simulink model "MSBR_Plant"  (R2021b)
settings: Solver=ode45  StartTime=0.0  StopTime=sim_time  MaxStep=ts_max  RelTol=1e-4
values from neighbouring files (symbols this model uses):
  a_1 = 8.7292e-2/wilson_ratio    (= 0.0087292)    [Whole_Plant_Cool_Pump_Accident_script.m]    (also in Whole_Plant_Fert_Pump_Accident_script.m; Whole_Plant_Fuel_Pump_Accident.m; Whole_Plant_Fuel_Pump_Accident_script.m; Whole_Plant_Reactivity_Accident.m)
  a_2 = 7.3787e-4/wilson_ratio    (= 7.3787e-05)    [Whole_Plant_Cool_Pump_Accident_script.m]    (also in Whole_Plant_Fert_Pump_Accident_script.m; Whole_Plant_Fuel_Pump_Accident.m; Whole_Plant_Fuel_Pump_Accident_script.m; Whole_Plant_Reactivity_Accident.m)
  a_b = 1.656e-5    (= 1.656e-05)    [Whole_Plant_Cool_Pump_Accident_script.m]    (also in Whole_Plant_Fert_Pump_Accident_script.m; Whole_Plant_Fuel_Pump_Accident.m; Whole_Plant_Fuel_Pump_Accident_script.m; Whole_Plant_Reactivity_Accident.m)
  a_f = -8.172e-5    (= -8.172e-05)    [Whole_Plant_Cool_Pump_Accident_script.m]    (also in Whole_Plant_Fert_Pump_Accident_script.m; Whole_Plant_Fuel_Pump_Accident.m; Whole_Plant_Fuel_Pump_Accident_script.m; Whole_Plant_Reactivity_Accident.m)
  a_g = 2.016e-5    (= 2.016e-05)    [Whole_Plant_Cool_Pump_Accident_script.m]    (also in Whole_Plant_Fert_Pump_Accident_script.m; Whole_Plant_Fuel_Pump_Accident.m; Whole_Plant_Fuel_Pump_Accident_script.m; Whole_Plant_Reactivity_Accident.m)
  A_s = pi()*((D_OTSG_i^2)/4) - A_w_OTSG - A_p_OTSG    [Whole_Plant_Cool_Pump_Accident_script.m]    (also in Whole_Plant_Fert_Pump_Accident_script.m; Whole_Plant_Fuel_Pump_Accident.m; Whole_Plant_Fuel_Pump_Accident_script.m; Whole_Plant_Reactivity_Accident.m)
  alpha_co = 316.2    [Whole_Plant_Cool_Pump_Accident_script.m]    (also in Whole_Plant_Fert_Pump_Accident_script.m; Whole_Plant_Fuel_Pump_Accident.m; Whole_Plant_Fuel_Pump_Accident_script.m; Whole_Plant_Reactivity_Accident.m)
  beta = [2.290e-04, 8.320e-04, 7.100e-04, 8.520e-04, 1.710e-04, 1.020e-04]    [Whole_Plant_Cool_Pump_Accident_script.m]    (also in Whole_Plant_Fert_Pump_Accident_script.m; Whole_Plant_Fuel_Pump_Accident.m; Whole_Plant_Fuel_Pump_Accident_script.m; Whole_Plant_Reactivity_Accident.m)
  beta_co = 68.0958    [Whole_Plant_Cool_Pump_Accident_script.m]    (also in Whole_Plant_Fert_Pump_Accident_script.m; Whole_Plant_Fuel_Pump_Accident.m; Whole_Plant_Fuel_Pump_Accident_script.m; Whole_Plant_Reactivity_Accident.m)
  beta_t = sum(beta)    [Whole_Plant_Cool_Pump_Accident_script.m]    (also in Whole_Plant_Fert_Pump_Accident_script.m; Whole_Plant_Fuel_Pump_Accident.m; Whole_Plant_Fuel_Pump_Accident_script.m; Whole_Plant_Reactivity_Accident.m)
  C_nc_X_A_nc = 12.8    [Whole_Plant_Cool_Pump_Accident_script.m]    (also in Whole_Plant_Fert_Pump_Accident_script.m; Whole_Plant_Fuel_Pump_Accident.m; Whole_Plant_Fuel_Pump_Accident_script.m; Whole_Plant_Reactivity_Accident.m)
  C_pcw = 0.0042    [Whole_Plant_Cool_Pump_Accident_script.m]    (also in Whole_Plant_Fert_Pump_Accident_script.m; Whole_Plant_Fuel_Pump_Accident.m; Whole_Plant_Fuel_Pump_Accident_script.m; Whole_Plant_Reactivity_Accident.m)
  C_rh_X_A_rh = 33    [Whole_Plant_Cool_Pump_Accident_script.m]    (also in Whole_Plant_Fert_Pump_Accident_script.m; Whole_Plant_Fuel_Pump_Accident.m; Whole_Plant_Fuel_Pump_Accident_script.m; Whole_Plant_Reactivity_Accident.m)
  C_v = 0.84    [Whole_Plant_Cool_Pump_Accident_script.m]    (also in Whole_Plant_Fert_Pump_Accident_script.m; Whole_Plant_Fuel_Pump_Accident.m; Whole_Plant_Fuel_Pump_Accident_script.m; Whole_Plant_Reactivity_Accident.m)
  ce1 = 1.2471e-07    [Whole_Plant_Cool_Pump_Accident_script.m]    (also in Whole_Plant_Fert_Pump_Accident_script.m; Whole_Plant_Fuel_Pump_Accident.m; Whole_Plant_Fuel_Pump_Accident_script.m; Whole_Plant_Reactivity_Accident.m)
  ce2 = 5.3816e-14    [Whole_Plant_Cool_Pump_Accident_script.m]    (also in Whole_Plant_Fert_Pump_Accident_script.m; Whole_Plant_Fuel_Pump_Accident.m; Whole_Plant_Fuel_Pump_Accident_script.m; Whole_Plant_Reactivity_Accident.m)
  ce3 = 3.3721e-08    [Whole_Plant_Cool_Pump_Accident_script.m]    (also in Whole_Plant_Fert_Pump_Accident_script.m; Whole_Plant_Fuel_Pump_Accident.m; Whole_Plant_Fuel_Pump_Accident_script.m; Whole_Plant_Reactivity_Accident.m)
  Cp_fw = XSteam('Cp_pT',P_set*10,T_fw)/1000    [Whole_Plant_Cool_Pump_Accident_script.m]    (also in Whole_Plant_Fert_Pump_Accident_script.m; Whole_Plant_Fuel_Pump_Accident.m; Whole_Plant_Fuel_Pump_Accident_script.m; Whole_Plant_Reactivity_Accident.m)
  Cp_p = Cp_sec    (= 0.001716588)    [Whole_Plant_Cool_Pump_Accident_script.m]    (also in Whole_Plant_Fert_Pump_Accident_script.m; Whole_Plant_Fuel_Pump_Accident.m; Whole_Plant_Fuel_Pump_Accident_script.m; Whole_Plant_Reactivity_Accident.m)
  Cp_rh = 0.0021520    (= 0.002152)    [Whole_Plant_Cool_Pump_Accident_script.m]    (also in Whole_Plant_Fert_Pump_Accident_script.m; Whole_Plant_Fuel_Pump_Accident.m; Whole_Plant_Fuel_Pump_Accident_script.m; Whole_Plant_Reactivity_Accident.m)
  Cp_s = XSteam('Cp_pT',P_s*10,T_s)/1000    [Whole_Plant_Cool_Pump_Accident_script.m]    (also in Whole_Plant_Fert_Pump_Accident_script.m; Whole_Plant_Fuel_Pump_Accident.m; Whole_Plant_Fuel_Pump_Accident_script.m; Whole_Plant_Reactivity_Accident.m)
  Cp_sc = XSteam('Cp_pT',P_set*10,T_sc2)/1000    [Whole_Plant_Cool_Pump_Accident_script.m]    (also in Whole_Plant_Fert_Pump_Accident_script.m; Whole_Plant_Fuel_Pump_Accident.m; Whole_Plant_Fuel_Pump_Accident_script.m; Whole_Plant_Reactivity_Accident.m)
  Cp_w = 468.992e-6    (= 0.000468992)    [Whole_Plant_Cool_Pump_Accident_script.m]    (also in Whole_Plant_Fert_Pump_Accident_script.m; Whole_Plant_Fuel_Pump_Accident.m; Whole_Plant_Fuel_Pump_Accident_script.m; Whole_Plant_Reactivity_Accident.m)
  D_it = D_ot-2*T_th    (= 0.014147)    [Whole_Plant_Cool_Pump_Accident_script.m]    (also in Whole_Plant_Fert_Pump_Accident_script.m; Whole_Plant_Fuel_Pump_Accident.m; Whole_Plant_Fuel_Pump_Accident_script.m; Whole_Plant_Reactivity_Accident.m)
  D_ot = 0.015875    [Whole_Plant_Cool_Pump_Accident_script.m]    (also in Whole_Plant_Fert_Pump_Accident_script.m; Whole_Plant_Fuel_Pump_Accident.m; Whole_Plant_Fuel_Pump_Accident_script.m; Whole_Plant_Reactivity_Accident.m)
  dHs_dPs = c(1)    [Whole_Plant_Cool_Pump_Accident_script.m]    (also in Whole_Plant_Fert_Pump_Accident_script.m; Whole_Plant_Fuel_Pump_Accident.m; Whole_Plant_Fuel_Pump_Accident_script.m; Whole_Plant_Reactivity_Accident.m)
  eta_hp_isen = 0.861    [Whole_Plant_Cool_Pump_Accident_script.m]    (also in Whole_Plant_Fert_Pump_Accident_script.m; Whole_Plant_Fuel_Pump_Accident.m; Whole_Plant_Fuel_Pump_Accident_script.m; Whole_Plant_Reactivity_Accident.m)
  eta_lp_isen = 0.861    [Whole_Plant_Cool_Pump_Accident_script.m]    (also in Whole_Plant_Fert_Pump_Accident_script.m; Whole_Plant_Fuel_Pump_Accident.m; Whole_Plant_Fuel_Pump_Accident_script.m; Whole_Plant_Reactivity_Accident.m)
  gamma_I = 5.1135e-2    (= 0.051135)    [Whole_Plant_Cool_Pump_Accident_script.m]    (also in Whole_Plant_Fert_Pump_Accident_script.m; Whole_Plant_Fuel_Pump_Accident.m; Whole_Plant_Fuel_Pump_Accident_script.m; Whole_Plant_Reactivity_Accident.m)
  gamma_Xe = 1.1628e-2    (= 0.011628)    [Whole_Plant_Cool_Pump_Accident_script.m]    (also in Whole_Plant_Fert_Pump_Accident_script.m; Whole_Plant_Fuel_Pump_Accident.m; Whole_Plant_Fuel_Pump_Accident_script.m; Whole_Plant_Reactivity_Accident.m)
  H_co0 = 0.149    [Whole_Plant_Cool_Pump_Accident_script.m]    (also in Whole_Plant_Fert_Pump_Accident_script.m; Whole_Plant_Fuel_Pump_Accident.m; Whole_Plant_Fuel_Pump_Accident_script.m; Whole_Plant_Reactivity_Accident.m)
  H_f_co0 = 0.149    [Whole_Plant_Cool_Pump_Accident_script.m]    (also in Whole_Plant_Fert_Pump_Accident_script.m; Whole_Plant_Fuel_Pump_Accident.m; Whole_Plant_Fuel_Pump_Accident_script.m; Whole_Plant_Reactivity_Accident.m)
  H_fg_co0 = 2.35    [Whole_Plant_Cool_Pump_Accident_script.m]    (also in Whole_Plant_Fert_Pump_Accident_script.m; Whole_Plant_Fuel_Pump_Accident.m; Whole_Plant_Fuel_Pump_Accident_script.m; Whole_Plant_Reactivity_Accident.m)
  H_fgrh0 = (XSteam('hV_p', P_s*1e1) - XSteam('hL_p', P_s*1e1))/1e3    [Whole_Plant_Cool_Pump_Accident_script.m]    (also in Whole_Plant_Fert_Pump_Accident_script.m; Whole_Plant_Fuel_Pump_Accident.m; Whole_Plant_Fuel_Pump_Accident_script.m; Whole_Plant_Reactivity_Accident.m)
  H_frh0 = XSteam('hL_p', P_s*1e1)/1e3    [Whole_Plant_Cool_Pump_Accident_script.m]    (also in Whole_Plant_Fert_Pump_Accident_script.m; Whole_Plant_Fuel_Pump_Accident.m; Whole_Plant_Fuel_Pump_Accident_script.m; Whole_Plant_Reactivity_Accident.m)
  h_fwh1 = 0.5927    [Whole_Plant_Cool_Pump_Accident_script.m]    (also in Whole_Plant_Fert_Pump_Accident_script.m; Whole_Plant_Fuel_Pump_Accident.m; Whole_Plant_Fuel_Pump_Accident_script.m; Whole_Plant_Reactivity_Accident.m)
  H_fwh10 = 0.46009    [Whole_Plant_Cool_Pump_Accident_script.m]    (also in Whole_Plant_Fert_Pump_Accident_script.m; Whole_Plant_Fuel_Pump_Accident.m; Whole_Plant_Fuel_Pump_Accident_script.m; Whole_Plant_Reactivity_Accident.m)
  h_fwh2 = 1.230803    [Whole_Plant_Cool_Pump_Accident_script.m]    (also in Whole_Plant_Fert_Pump_Accident_script.m; Whole_Plant_Fuel_Pump_Accident.m; Whole_Plant_Fuel_Pump_Accident_script.m; Whole_Plant_Reactivity_Accident.m)
  H_fwh20 = 0.6784    [Whole_Plant_Cool_Pump_Accident_script.m]    (also in Whole_Plant_Fert_Pump_Accident_script.m; Whole_Plant_Fuel_Pump_Accident.m; Whole_Plant_Fuel_Pump_Accident_script.m; Whole_Plant_Reactivity_Accident.m)
  H_grh0 = 2.8029    [Whole_Plant_Cool_Pump_Accident_script.m]    (also in Whole_Plant_Fert_Pump_Accident_script.m; Whole_Plant_Fuel_Pump_Accident.m; Whole_Plant_Fuel_Pump_Accident_script.m; Whole_Plant_Reactivity_Accident.m)
  H_hp_isen0 = 2.5111    [Whole_Plant_Cool_Pump_Accident_script.m]    (also in Whole_Plant_Fert_Pump_Accident_script.m; Whole_Plant_Fuel_Pump_Accident.m; Whole_Plant_Fuel_Pump_Accident_script.m; Whole_Plant_Reactivity_Accident.m)
  H_hpt_out = 2.6201    [Whole_Plant_Cool_Pump_Accident_script.m]    (also in Whole_Plant_Fert_Pump_Accident_script.m; Whole_Plant_Fuel_Pump_Accident.m; Whole_Plant_Fuel_Pump_Accident_script.m; Whole_Plant_Reactivity_Accident.m)
  H_lp_isen = 958.4*1054.35e-6/0.45359237    (= 2.22774699671)    [Whole_Plant_Cool_Pump_Accident_script.m]    (also in Whole_Plant_Fert_Pump_Accident_script.m; Whole_Plant_Fuel_Pump_Accident.m; Whole_Plant_Fuel_Pump_Accident_script.m; Whole_Plant_Reactivity_Accident.m)
  H_lpt_out = 2.3089    [Whole_Plant_Cool_Pump_Accident_script.m]    (also in Whole_Plant_Fert_Pump_Accident_script.m; Whole_Plant_Fuel_Pump_Accident.m; Whole_Plant_Fuel_Pump_Accident_script.m; Whole_Plant_Reactivity_Accident.m)
  H_nc = XSteam('h_pT', P_s*10, T_s)/1000    [Whole_Plant_Cool_Pump_Accident_script.m]    (also in Whole_Plant_Fert_Pump_Accident_script.m; Whole_Plant_Fuel_Pump_Accident.m; Whole_Plant_Fuel_Pump_Accident_script.m; Whole_Plant_Reactivity_Accident.m)
  h_pw = h_s    (= 0.02555)    [Whole_Plant_Cool_Pump_Accident_script.m]    (also in Whole_Plant_Fert_Pump_Accident_script.m; Whole_Plant_Fuel_Pump_Accident.m; Whole_Plant_Fuel_Pump_Accident_script.m; Whole_Plant_Reactivity_Accident.m)
  H_rh = 2.8115    [Whole_Plant_Cool_Pump_Accident_script.m]    (also in Whole_Plant_Fert_Pump_Accident_script.m; Whole_Plant_Fuel_Pump_Accident.m; Whole_Plant_Fuel_Pump_Accident_script.m; Whole_Plant_Reactivity_Accident.m)
  h_wb = 13349.334646671E-6    (= 0.0133493346467)    [Whole_Plant_Cool_Pump_Accident_script.m]    (also in Whole_Plant_Fert_Pump_Accident_script.m; Whole_Plant_Fuel_Pump_Accident.m; Whole_Plant_Fuel_Pump_Accident_script.m; Whole_Plant_Reactivity_Accident.m)
  h_ws = 5732.378387768E-6    (= 0.00573237838777)    [Whole_Plant_Cool_Pump_Accident_script.m]    (also in Whole_Plant_Fert_Pump_Accident_script.m; Whole_Plant_Fuel_Pump_Accident.m; Whole_Plant_Fuel_Pump_Accident_script.m; Whole_Plant_Reactivity_Accident.m)
  h_wsc = 8385.005556375E-6    (= 0.00838500555638)    [Whole_Plant_Cool_Pump_Accident_script.m]    (also in Whole_Plant_Fert_Pump_Accident_script.m; Whole_Plant_Fuel_Pump_Accident.m; Whole_Plant_Fuel_Pump_Accident_script.m; Whole_Plant_Reactivity_Accident.m)
  hA_bg = A_fert*h_bg    (= 2.76411813627)    [Whole_Plant_Cool_Pump_Accident_script.m]    (also in Whole_Plant_Fert_Pump_Accident_script.m; Whole_Plant_Fuel_Pump_Accident.m; Whole_Plant_Fuel_Pump_Accident_script.m; Whole_Plant_Reactivity_Accident.m)
  hA_co0 = 140    [Whole_Plant_Cool_Pump_Accident_script.m]    (also in Whole_Plant_Fert_Pump_Accident_script.m; Whole_Plant_Fuel_Pump_Accident.m; Whole_Plant_Fuel_Pump_Accident_script.m; Whole_Plant_Reactivity_Accident.m)
  hA_fg_dn = h_fg*A_fuel_down    [Whole_Plant_Cool_Pump_Accident_script.m]    (also in Whole_Plant_Fert_Pump_Accident_script.m; Whole_Plant_Fuel_Pump_Accident.m; Whole_Plant_Fuel_Pump_Accident_script.m; Whole_Plant_Reactivity_Accident.m)
  hA_fg_up = h_fg*A_fuel_up    [Whole_Plant_Cool_Pump_Accident_script.m]    (also in Whole_Plant_Fert_Pump_Accident_script.m; Whole_Plant_Fuel_Pump_Accident.m; Whole_Plant_Fuel_Pump_Accident_script.m; Whole_Plant_Reactivity_Accident.m)
  hA_p_bhx1 = [h_pb*A_pbhx/2,h_pb*A_pbhx/2]    [Whole_Plant_Cool_Pump_Accident_script.m]    (also in Whole_Plant_Fert_Pump_Accident_script.m; Whole_Plant_Fuel_Pump_Accident.m; Whole_Plant_Fuel_Pump_Accident_script.m; Whole_Plant_Reactivity_Accident.m)
  hA_p_bhx2 = hA_p_bhx1    [Whole_Plant_Cool_Pump_Accident_script.m]    (also in Whole_Plant_Fert_Pump_Accident_script.m; Whole_Plant_Fuel_Pump_Accident.m; Whole_Plant_Fuel_Pump_Accident_script.m; Whole_Plant_Reactivity_Accident.m)
  hA_p_bhx3 = hA_p_bhx1    [Whole_Plant_Cool_Pump_Accident_script.m]    (also in Whole_Plant_Fert_Pump_Accident_script.m; Whole_Plant_Fuel_Pump_Accident.m; Whole_Plant_Fuel_Pump_Accident_script.m; Whole_Plant_Reactivity_Accident.m)
  hA_p_bhx4 = hA_p_bhx1    [Whole_Plant_Cool_Pump_Accident_script.m]    (also in Whole_Plant_Fert_Pump_Accident_script.m; Whole_Plant_Fuel_Pump_Accident.m; Whole_Plant_Fuel_Pump_Accident_script.m; Whole_Plant_Reactivity_Accident.m)
  hA_p_fhx1 = [h_p*A_pfhx_dn/2,h_p*A_pfhx_dn/2,h_p*A_pfhx_up/2,h_p*A_pfhx_up/2]    [Whole_Plant_Cool_Pump_Accident_script.m]    (also in Whole_Plant_Fert_Pump_Accident_script.m; Whole_Plant_Fuel_Pump_Accident.m; Whole_Plant_Fuel_Pump_Accident_script.m; Whole_Plant_Reactivity_Accident.m)
  hA_p_fhx2 = hA_p_fhx1    [Whole_Plant_Cool_Pump_Accident_script.m]    (also in Whole_Plant_Fert_Pump_Accident_script.m; Whole_Plant_Fuel_Pump_Accident.m; Whole_Plant_Fuel_Pump_Accident_script.m; Whole_Plant_Reactivity_Accident.m)
  hA_p_fhx3 = hA_p_fhx1    [Whole_Plant_Cool_Pump_Accident_script.m]    (also in Whole_Plant_Fert_Pump_Accident_script.m; Whole_Plant_Fuel_Pump_Accident.m; Whole_Plant_Fuel_Pump_Accident_script.m; Whole_Plant_Reactivity_Accident.m)
  hA_p_fhx4 = hA_p_fhx1    [Whole_Plant_Cool_Pump_Accident_script.m]    (also in Whole_Plant_Fert_Pump_Accident_script.m; Whole_Plant_Fuel_Pump_Accident.m; Whole_Plant_Fuel_Pump_Accident_script.m; Whole_Plant_Reactivity_Accident.m)
  hA_s_bhx1 = [h_sb*A_sbhx/2,h_sb*A_sbhx/2]    [Whole_Plant_Cool_Pump_Accident_script.m]    (also in Whole_Plant_Fert_Pump_Accident_script.m; Whole_Plant_Fuel_Pump_Accident.m; Whole_Plant_Fuel_Pump_Accident_script.m; Whole_Plant_Reactivity_Accident.m)
  hA_s_bhx2 = hA_s_bhx1    [Whole_Plant_Cool_Pump_Accident_script.m]    (also in Whole_Plant_Fert_Pump_Accident_script.m; Whole_Plant_Fuel_Pump_Accident.m; Whole_Plant_Fuel_Pump_Accident_script.m; Whole_Plant_Reactivity_Accident.m)
  hA_s_bhx3 = hA_s_bhx1    [Whole_Plant_Cool_Pump_Accident_script.m]    (also in Whole_Plant_Fert_Pump_Accident_script.m; Whole_Plant_Fuel_Pump_Accident.m; Whole_Plant_Fuel_Pump_Accident_script.m; Whole_Plant_Reactivity_Accident.m)
  hA_s_bhx4 = hA_s_bhx1    [Whole_Plant_Cool_Pump_Accident_script.m]    (also in Whole_Plant_Fert_Pump_Accident_script.m; Whole_Plant_Fuel_Pump_Accident.m; Whole_Plant_Fuel_Pump_Accident_script.m; Whole_Plant_Reactivity_Accident.m)
  hA_s_fhx1 = [h_s*A_sfhx_up/2,h_s*A_sfhx_up/2,h_s*A_sfhx_dn/2,h_s*A_sfhx_dn/2]    [Whole_Plant_Cool_Pump_Accident_script.m]    (also in Whole_Plant_Fert_Pump_Accident_script.m; Whole_Plant_Fuel_Pump_Accident.m; Whole_Plant_Fuel_Pump_Accident_script.m; Whole_Plant_Reactivity_Accident.m)
  hA_s_fhx2 = hA_s_fhx1    [Whole_Plant_Cool_Pump_Accident_script.m]    (also in Whole_Plant_Fert_Pump_Accident_script.m; Whole_Plant_Fuel_Pump_Accident.m; Whole_Plant_Fuel_Pump_Accident_script.m; Whole_Plant_Reactivity_Accident.m)
  hA_s_fhx3 = hA_s_fhx1    [Whole_Plant_Cool_Pump_Accident_script.m]    (also in Whole_Plant_Fert_Pump_Accident_script.m; Whole_Plant_Fuel_Pump_Accident.m; Whole_Plant_Fuel_Pump_Accident_script.m; Whole_Plant_Reactivity_Accident.m)
  hA_s_fhx4 = hA_s_fhx1    [Whole_Plant_Cool_Pump_Accident_script.m]    (also in Whole_Plant_Fert_Pump_Accident_script.m; Whole_Plant_Fuel_Pump_Accident.m; Whole_Plant_Fuel_Pump_Accident_script.m; Whole_Plant_Reactivity_Accident.m)
  I_0 = gamma_I*Sigma_f_msbr*phi_0/lam_I    (= 1.30000734126e+17)    [Whole_Plant_Cool_Pump_Accident_script.m]    (also in Whole_Plant_Fert_Pump_Accident_script.m; Whole_Plant_Fuel_Pump_Accident.m; Whole_Plant_Fuel_Pump_Accident_script.m; Whole_Plant_Reactivity_Accident.m)
  k_1 = 0.5    [Whole_Plant_Cool_Pump_Accident_script.m]    (also in Whole_Plant_Fert_Pump_Accident_script.m; Whole_Plant_Fuel_Pump_Accident.m; Whole_Plant_Fuel_Pump_Accident_script.m; Whole_Plant_Reactivity_Accident.m)
  K_1 = e(1)    [Whole_Plant_Cool_Pump_Accident_script.m]    (also in Whole_Plant_Fert_Pump_Accident_script.m; Whole_Plant_Fuel_Pump_Accident.m; Whole_Plant_Fuel_Pump_Accident_script.m; Whole_Plant_Reactivity_Accident.m)
  k_1b = 0.5    [Whole_Plant_Cool_Pump_Accident_script.m]    (also in Whole_Plant_Fert_Pump_Accident_script.m; Whole_Plant_Fuel_Pump_Accident.m; Whole_Plant_Fuel_Pump_Accident_script.m; Whole_Plant_Reactivity_Accident.m)
  k_2 = 0.5    [Whole_Plant_Cool_Pump_Accident_script.m]    (also in Whole_Plant_Fert_Pump_Accident_script.m; Whole_Plant_Fuel_Pump_Accident.m; Whole_Plant_Fuel_Pump_Accident_script.m; Whole_Plant_Reactivity_Accident.m)
  k_2b = 0.5    [Whole_Plant_Cool_Pump_Accident_script.m]    (also in Whole_Plant_Fert_Pump_Accident_script.m; Whole_Plant_Fuel_Pump_Accident.m; Whole_Plant_Fuel_Pump_Accident_script.m; Whole_Plant_Reactivity_Accident.m)
  k_3 = 0.5    [Whole_Plant_Cool_Pump_Accident_script.m]    (also in Whole_Plant_Fert_Pump_Accident_script.m; Whole_Plant_Fuel_Pump_Accident.m; Whole_Plant_Fuel_Pump_Accident_script.m; Whole_Plant_Reactivity_Accident.m)
  k_4 = 0.5    [Whole_Plant_Cool_Pump_Accident_script.m]    (also in Whole_Plant_Fert_Pump_Accident_script.m; Whole_Plant_Fuel_Pump_Accident.m; Whole_Plant_Fuel_Pump_Accident_script.m; Whole_Plant_Reactivity_Accident.m)
  K_4 = b(1)    [Whole_Plant_Cool_Pump_Accident_script.m]    (also in Whole_Plant_Fert_Pump_Accident_script.m; Whole_Plant_Fuel_Pump_Accident.m; Whole_Plant_Fuel_Pump_Accident_script.m; Whole_Plant_Reactivity_Accident.m)
  K_5 = a(1)    [Whole_Plant_Cool_Pump_Accident_script.m]    (also in Whole_Plant_Fert_Pump_Accident_script.m; Whole_Plant_Fuel_Pump_Accident.m; Whole_Plant_Fuel_Pump_Accident_script.m; Whole_Plant_Reactivity_Accident.m)
  K_b = d(1)    [Whole_Plant_Cool_Pump_Accident_script.m]    (also in Whole_Plant_Fert_Pump_Accident_script.m; Whole_Plant_Fuel_Pump_Accident.m; Whole_Plant_Fuel_Pump_Accident_script.m; Whole_Plant_Reactivity_Accident.m)
  k_b1 = (K_B/2)/K    (= 0.0089463103122)    [Whole_Plant_Cool_Pump_Accident_script.m]    (also in Whole_Plant_Fert_Pump_Accident_script.m; Whole_Plant_Fuel_Pump_Accident.m; Whole_Plant_Fuel_Pump_Accident_script.m; Whole_Plant_Reactivity_Accident.m)
  k_b2 = k_b1    (= 0.0089463103122)    [Whole_Plant_Cool_Pump_Accident_script.m]    (also in Whole_Plant_Fert_Pump_Accident_script.m; Whole_Plant_Fuel_Pump_Accident.m; Whole_Plant_Fuel_Pump_Accident_script.m; Whole_Plant_Reactivity_Accident.m)
  K_bhp = 0.1634    [Whole_Plant_Cool_Pump_Accident_script.m]    (also in Whole_Plant_Fert_Pump_Accident_script.m; Whole_Plant_Fuel_Pump_Accident.m; Whole_Plant_Fuel_Pump_Accident_script.m; Whole_Plant_Reactivity_Accident.m)
  K_blp = 0.2174    [Whole_Plant_Cool_Pump_Accident_script.m]    (also in Whole_Plant_Fert_Pump_Accident_script.m; Whole_Plant_Fuel_Pump_Accident.m; Whole_Plant_Fuel_Pump_Accident_script.m; Whole_Plant_Reactivity_Accident.m)
  k_f1 = ((1 - K_G - K_B - K_Ba)/4)/K    (= 0.226055463576)    [Whole_Plant_Cool_Pump_Accident_script.m]    (also in Whole_Plant_Fert_Pump_Accident_script.m; Whole_Plant_Fuel_Pump_Accident.m; Whole_Plant_Fuel_Pump_Accident_script.m; Whole_Plant_Reactivity_Accident.m)
  k_f2 = k_f1    (= 0.226055463576)    [Whole_Plant_Cool_Pump_Accident_script.m]    (also in Whole_Plant_Fert_Pump_Accident_script.m; Whole_Plant_Fuel_Pump_Accident.m; Whole_Plant_Fuel_Pump_Accident_script.m; Whole_Plant_Reactivity_Accident.m)
  k_f3 = k_f1    (= 0.226055463576)    [Whole_Plant_Cool_Pump_Accident_script.m]    (also in Whole_Plant_Fert_Pump_Accident_script.m; Whole_Plant_Fuel_Pump_Accident.m; Whole_Plant_Fuel_Pump_Accident_script.m; Whole_Plant_Reactivity_Accident.m)
  k_f4 = k_f1    (= 0.226055463576)    [Whole_Plant_Cool_Pump_Accident_script.m]    (also in Whole_Plant_Fert_Pump_Accident_script.m; Whole_Plant_Fuel_Pump_Accident.m; Whole_Plant_Fuel_Pump_Accident_script.m; Whole_Plant_Reactivity_Accident.m)
  k_g1 = ((K_G*K_fuel)/2)/K    (= 0.0346590586566)    [Whole_Plant_Cool_Pump_Accident_script.m]    (also in Whole_Plant_Fert_Pump_Accident_script.m; Whole_Plant_Fuel_Pump_Accident.m; Whole_Plant_Fuel_Pump_Accident_script.m; Whole_Plant_Reactivity_Accident.m)
  k_g2 = k_g1    (= 0.0346590586566)    [Whole_Plant_Cool_Pump_Accident_script.m]    (also in Whole_Plant_Fert_Pump_Accident_script.m; Whole_Plant_Fuel_Pump_Accident.m; Whole_Plant_Fuel_Pump_Accident_script.m; Whole_Plant_Reactivity_Accident.m)
  k_g3 = (K_G*(1-K_fuel))/K    (= 0.00856740775781)    [Whole_Plant_Cool_Pump_Accident_script.m]    (also in Whole_Plant_Fert_Pump_Accident_script.m; Whole_Plant_Fuel_Pump_Accident.m; Whole_Plant_Fuel_Pump_Accident_script.m; Whole_Plant_Reactivity_Accident.m)
  K_sc = f(1)    [Whole_Plant_Cool_Pump_Accident_script.m]    (also in Whole_Plant_Fert_Pump_Accident_script.m; Whole_Plant_Fuel_Pump_Accident.m; Whole_Plant_Fuel_Pump_Accident_script.m; Whole_Plant_Reactivity_Accident.m)
  L = 22.0    (= 22)    [Whole_Plant_Cool_Pump_Accident_script.m]    (also in Whole_Plant_Fert_Pump_Accident_script.m; Whole_Plant_Fuel_Pump_Accident.m; Whole_Plant_Fuel_Pump_Accident_script.m; Whole_Plant_Reactivity_Accident.m)
  L_b = 1.9    [Whole_Plant_Cool_Pump_Accident_script.m]    (also in Whole_Plant_Fert_Pump_Accident_script.m; Whole_Plant_Fuel_Pump_Accident.m; Whole_Plant_Fuel_Pump_Accident_script.m; Whole_Plant_Reactivity_Accident.m)
  L_s = 16.53    [Whole_Plant_Cool_Pump_Accident_script.m]    (also in Whole_Plant_Fert_Pump_Accident_script.m; Whole_Plant_Fuel_Pump_Accident.m; Whole_Plant_Fuel_Pump_Accident_script.m; Whole_Plant_Reactivity_Accident.m)
  L_sc = L-L_b-L_s    (= 3.57)    [Whole_Plant_Cool_Pump_Accident_script.m]    (also in Whole_Plant_Fert_Pump_Accident_script.m; Whole_Plant_Fuel_Pump_Accident.m; Whole_Plant_Fuel_Pump_Accident_script.m; Whole_Plant_Reactivity_Accident.m)
  Lam = 3.3e-4    (= 0.00033)    [Whole_Plant_Cool_Pump_Accident_script.m]    (also in Whole_Plant_Fert_Pump_Accident_script.m; Whole_Plant_Fuel_Pump_Accident.m; Whole_Plant_Fuel_Pump_Accident_script.m; Whole_Plant_Reactivity_Accident.m)
  lam = [1.260e-02, 3.370e-02, 1.390e-01, 3.250e-01, 1.130e+00, 2.500e+00]    [Whole_Plant_Cool_Pump_Accident_script.m]    (also in Whole_Plant_Fert_Pump_Accident_script.m; Whole_Plant_Fuel_Pump_Accident.m; Whole_Plant_Fuel_Pump_Accident_script.m; Whole_Plant_Reactivity_Accident.m)
  lam_bubl = 2.0e-2    (= 0.02)    [Whole_Plant_Cool_Pump_Accident_script.m]    (also in Whole_Plant_Fert_Pump_Accident_script.m; Whole_Plant_Fuel_Pump_Accident.m; Whole_Plant_Fuel_Pump_Accident_script.m; Whole_Plant_Reactivity_Accident.m)
  lam_I = 2.875e-5    (= 2.875e-05)    [Whole_Plant_Cool_Pump_Accident_script.m]    (also in Whole_Plant_Fert_Pump_Accident_script.m; Whole_Plant_Fuel_Pump_Accident.m; Whole_Plant_Fuel_Pump_Accident_script.m; Whole_Plant_Reactivity_Accident.m)
  lam_Xe = 2.0916e-5    (= 2.0916e-05)    [Whole_Plant_Cool_Pump_Accident_script.m]    (also in Whole_Plant_Fert_Pump_Accident_script.m; Whole_Plant_Fuel_Pump_Accident.m; Whole_Plant_Fuel_Pump_Accident_script.m; Whole_Plant_Reactivity_Accident.m)
  m_bm = (W_b1+W_b2+W_b3+W_b4)*time_mixb    (= 2167.1636)    [Whole_Plant_Cool_Pump_Accident_script.m]    (also in Whole_Plant_Fert_Pump_Accident_script.m; Whole_Plant_Fuel_Pump_Accident.m; Whole_Plant_Fuel_Pump_Accident_script.m; Whole_Plant_Reactivity_Accident.m)
  M_cw = 65000    [Whole_Plant_Cool_Pump_Accident_script.m]    (also in Whole_Plant_Fert_Pump_Accident_script.m; Whole_Plant_Fuel_Pump_Accident.m; Whole_Plant_Fuel_Pump_Accident_script.m; Whole_Plant_Reactivity_Accident.m)
  m_fm = (W_f1+W_f2+W_f3+W_f4)*time_mixf    (= 5443.108)    [Whole_Plant_Cool_Pump_Accident_script.m]    (also in Whole_Plant_Fert_Pump_Accident_script.m; Whole_Plant_Fuel_Pump_Accident.m; Whole_Plant_Fuel_Pump_Accident_script.m; Whole_Plant_Reactivity_Accident.m)
  M_hw0 = 10000    [Whole_Plant_Cool_Pump_Accident_script.m]    (also in Whole_Plant_Fert_Pump_Accident_script.m; Whole_Plant_Fuel_Pump_Accident.m; Whole_Plant_Fuel_Pump_Accident_script.m; Whole_Plant_Reactivity_Accident.m)
  m_sm = (W_s1+W_s2+W_s3+W_s4)*time_mixs    (= 8467.056)    [Whole_Plant_Cool_Pump_Accident_script.m]    (also in Whole_Plant_Fert_Pump_Accident_script.m; Whole_Plant_Fuel_Pump_Accident.m; Whole_Plant_Fuel_Pump_Accident_script.m; Whole_Plant_Reactivity_Accident.m)
  M_stm = 0.018    [Whole_Plant_Cool_Pump_Accident_script.m]    (also in Whole_Plant_Fert_Pump_Accident_script.m; Whole_Plant_Fuel_Pump_Accident.m; Whole_Plant_Fuel_Pump_Accident_script.m; Whole_Plant_Reactivity_Accident.m)
  mcp_b1 = mass_bn*Cp_b    (= 4.17494922705)    [Whole_Plant_Cool_Pump_Accident_script.m]    (also in Whole_Plant_Fert_Pump_Accident_script.m; Whole_Plant_Fuel_Pump_Accident.m; Whole_Plant_Fuel_Pump_Accident_script.m; Whole_Plant_Reactivity_Accident.m)
  mcp_b2 = mcp_b1    (= 4.17494922705)    [Whole_Plant_Cool_Pump_Accident_script.m]    (also in Whole_Plant_Fert_Pump_Accident_script.m; Whole_Plant_Fuel_Pump_Accident.m; Whole_Plant_Fuel_Pump_Accident_script.m; Whole_Plant_Reactivity_Accident.m)
  mcp_f1 = mass_fn*Cp_f    (= 5.5019469141)    [Whole_Plant_Cool_Pump_Accident_script.m]    (also in Whole_Plant_Fert_Pump_Accident_script.m; Whole_Plant_Fuel_Pump_Accident.m; Whole_Plant_Fuel_Pump_Accident_script.m; Whole_Plant_Reactivity_Accident.m)
  mcp_f2 = mass_fn*Cp_f    (= 5.5019469141)    [Whole_Plant_Cool_Pump_Accident_script.m]    (also in Whole_Plant_Fert_Pump_Accident_script.m; Whole_Plant_Fuel_Pump_Accident.m; Whole_Plant_Fuel_Pump_Accident_script.m; Whole_Plant_Reactivity_Accident.m)
  mcp_f3 = mass_fn*Cp_f    (= 5.5019469141)    [Whole_Plant_Cool_Pump_Accident_script.m]    (also in Whole_Plant_Fert_Pump_Accident_script.m; Whole_Plant_Fuel_Pump_Accident.m; Whole_Plant_Fuel_Pump_Accident_script.m; Whole_Plant_Reactivity_Accident.m)
  mcp_f4 = mass_fn*Cp_f    (= 5.5019469141)    [Whole_Plant_Cool_Pump_Accident_script.m]    (also in Whole_Plant_Fert_Pump_Accident_script.m; Whole_Plant_Fuel_Pump_Accident.m; Whole_Plant_Fuel_Pump_Accident_script.m; Whole_Plant_Reactivity_Accident.m)
  mcp_g1 = (mass_grap*Cp_g)*K_fuel/2    (= 32.9814988203)    [Whole_Plant_Cool_Pump_Accident_script.m]    (also in Whole_Plant_Fert_Pump_Accident_script.m; Whole_Plant_Fuel_Pump_Accident.m; Whole_Plant_Fuel_Pump_Accident_script.m; Whole_Plant_Reactivity_Accident.m)
  mcp_g2 = mcp_g1    (= 32.9814988203)    [Whole_Plant_Cool_Pump_Accident_script.m]    (also in Whole_Plant_Fert_Pump_Accident_script.m; Whole_Plant_Fuel_Pump_Accident.m; Whole_Plant_Fuel_Pump_Accident_script.m; Whole_Plant_Reactivity_Accident.m)
  mcp_g3 = (mass_grap*Cp_g)*(1-K_fuel)    (= 8.15273004546)    [Whole_Plant_Cool_Pump_Accident_script.m]    (also in Whole_Plant_Fert_Pump_Accident_script.m; Whole_Plant_Fuel_Pump_Accident.m; Whole_Plant_Fuel_Pump_Accident_script.m; Whole_Plant_Reactivity_Accident.m)
  mcp_p_bhx1 = mp_bhx1*Cp_b    [Whole_Plant_Cool_Pump_Accident_script.m]    (also in Whole_Plant_Fert_Pump_Accident_script.m; Whole_Plant_Fuel_Pump_Accident.m; Whole_Plant_Fuel_Pump_Accident_script.m; Whole_Plant_Reactivity_Accident.m)
  mcp_p_bhx2 = mp_bhx2*Cp_b    [Whole_Plant_Cool_Pump_Accident_script.m]    (also in Whole_Plant_Fert_Pump_Accident_script.m; Whole_Plant_Fuel_Pump_Accident.m; Whole_Plant_Fuel_Pump_Accident_script.m; Whole_Plant_Reactivity_Accident.m)
  mcp_p_bhx3 = mp_bhx3*Cp_b    [Whole_Plant_Cool_Pump_Accident_script.m]    (also in Whole_Plant_Fert_Pump_Accident_script.m; Whole_Plant_Fuel_Pump_Accident.m; Whole_Plant_Fuel_Pump_Accident_script.m; Whole_Plant_Reactivity_Accident.m)
  ... (+213 more)
undefined symbols (not defined in the file or in its folder): C0, H_con_table, H_convap_table, H_rh_table, H_rh_table1, H_rh_table2, H_rhvap_table, H_s_table, H_table, P_con_table, P_nc_table, P_rh_table, P_rh_table1, pres_table, rho_rh_table, rho_table, SV_nc_table, SVf_nc_table, temp_table
(part 4 of 13)

== system MSBR_Plant/Nuclear Steam Supply System (NSSS)/Coolant Salt Pumps/Coolant Pump 4 ==
  note: Note that it is possible to put in a step function for the pump to reduce flow rate at a specific time. It could simulate a pipe leak/break
  note: Exponentional Function that decays with time (beginning at pump trip time). Decay rate is determined by tau_p of the pump. Final fractonal value of flow through piping is the thermal conv.
  Pump Decay Rate : Inport
  Thermal Conv : Inport  Port=2
  Pump Trip Time : Inport  Port=3
  1-D Lookup Table1 : Lookup_n-D  NumberOfTableDimensions=1  BreakpointsForDimension1=xdatc  Table=ydatc  InternalRulePriority=Speed  RndMeth=Simplest  InputSameDT=on
  Clock1 : Clock
  Constant : Constant
  Constant1 : Constant  Value=-1
  Divide : Product  Inputs=*/
  Math Function : Math  SaturateOnIntegerOverflow=on
  Minus : Sum  Inputs=+-
  Minus1 : Sum  Inputs=+-
  Minus3 : Sum  Inputs=+-
  Product : Product
  Scope1 : Scope
  Switch1 : Switch  Criteria=u2 > Threshold
  Switch3 : Switch  Criteria=u2 > Threshold
  To Workspace : ToWorkspace  VariableName=cool_pump_4_flow_frac  SaveFormat=Timeseries  SampleTime=-1
  To Workspace1 : ToWorkspace  VariableName=cool_pump_4_hA_frac  SaveFormat=Timeseries  SampleTime=-1
  Coolant Flow Fraction : Outport  VectorParamsAs1DForOutWhenUnconnected=off
  Coolant Heat Transfer Fraction : Outport  Port=2  VectorParamsAs1DForOutWhenUnconnected=off
  wires:
  Minus3/1 -> Switch3/2
  Product/1 -> Math Function/1
  Minus1/1 -> Product/1
  Divide/1 -> Product/2
  Constant1/1 -> Divide/1
  Constant/1 -> Switch1/1
  Clock1/1 -> Minus1/1, Minus/2
  Math Function/1 -> Switch1/3
  Switch1/1 -> Minus3/1, Switch3/1
  Minus/1 -> Switch1/2
  Pump Decay Rate/1 -> Divide/2
  Thermal Conv/1 -> Switch3/3, Minus3/2
  Pump Trip Time/1 -> Minus1/2, Minus/1
  Switch3/1 -> 1-D Lookup Table1/1, Scope1/1, To Workspace/1, Coolant Flow Fraction/1
  1-D Lookup Table1/1 -> To Workspace1/1, Coolant Heat Transfer Fraction/1

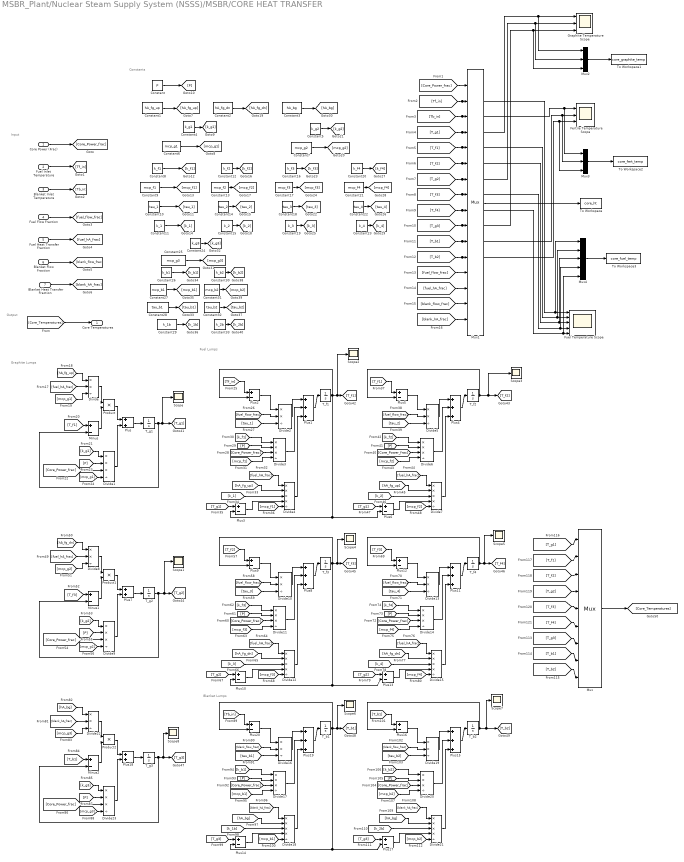
== system MSBR_Plant/Nuclear Steam Supply System (NSSS)/MSBR/CORE HEAT TRANSFER ==
  note: Constants
  note: Output
  note: Input
  note: Blanket Lumps
  note: Graphite Lumps
  note: Fuel Lumps
  Core Power (Frac) : Inport
  Fuel Inlet Temperature : Inport  Port=2
  Blanket Inlet Temperature : Inport  Port=3
  Fuel Flow Fraction : Inport  Port=4
  Fuel Heat Transfer Fraction : Inport  Port=5
  Blanket Flow Fraction : Inport  Port=6
  Blanket Heat Transfer Fraction : Inport  Port=7
  Constant : Constant  Value=P
  Constant1 : Constant  Value=hA_fg_up
  Constant10 : Constant  Value=tau_1
  Constant11 : Constant  Value=k_1
  Constant12 : Constant  Value=k_f2
  Constant13 : Constant  Value=mcp_f2
  Constant14 : Constant  Value=tau_2
  Constant15 : Constant  Value=k_2
  Constant16 : Constant  Value=k_f3
  Constant17 : Constant  Value=mcp_f3
  Constant18 : Constant  Value=tau_3
  Constant19 : Constant  Value=k_3
  Constant2 : Constant  Value=hA_fg_dn
  Constant20 : Constant  Value=k_f4
  Constant21 : Constant  Value=mcp_f4
  Constant22 : Constant  Value=tau_4
  Constant23 : Constant  Value=k_4
  Constant24 : Constant  Value=k_g3
  Constant25 : Constant  Value=mcp_g3
  Constant26 : Constant  Value=k_b1
  Constant27 : Constant  Value=mcp_b1
  Constant28 : Constant  Value=tau_b1
  Constant29 : Constant  Value=k_1b
  Constant3 : Constant  Value=hA_bg
  Constant30 : Constant  Value=k_b2
  Constant31 : Constant  Value=mcp_b2
  Constant32 : Constant  Value=tau_b2
  Constant33 : Constant  Value=k_2b
  Constant4 : Constant  Value=k_g1
  Constant5 : Constant  Value=k_g2
  Constant6 : Constant  Value=mcp_g1
  Constant7 : Constant  Value=mcp_g2
  Constant8 : Constant  Value=k_f1
  Constant9 : Constant  Value=mcp_f1
  Divide{,2,5,8,10,13,16,19,22} (9 alike) : Product  Inputs=**/
  Divide{1,3,6,9,11,14,17,20,23} (9 alike) : Product  Inputs=***/
  Divide{4,7,12,15,18,21} (6 alike) : Product  Inputs=****/
  Fertile Temperature Scope : Scope  NumInputPorts=3
  Fuel Temperature Scope : Scope  NumInputPorts=5
  Graphite Temperature Scope : Scope  NumInputPorts=3
  Minus : Sum  Inputs=+-
  Minus1 : Sum  Inputs=+-
  Minus2 : Sum  Inputs=+-
  Mux : Mux  Inputs=9
  Mux1 : Mux  Inputs=16
  Mux2 : Mux  Inputs=3
  Mux3 : Mux  Inputs=3
  Mux4 : Mux  Inputs=5
  Plus : Sum
  Plus{1,4,8,11,15,19} (6 alike) : Sum  Inputs=+++
  Plus{2..3,5..6,9..10,12..14,16..17,20} (12 alike) : Sum  Inputs=+-
  Plus18 : Sum
  Plus7 : Sum
  Product : Product
  Product1 : Product
  Product2 : Product
  Scope{,1..8} (9 alike) : Scope
  T_b1 : Integrator  InitialCondition=T0_b1
  T_b2 : Integrator  InitialCondition=T0_b2
  T_f1 : Integrator  InitialCondition=T0_f1
  T_f2 : Integrator  InitialCondition=T0_f2
  T_f3 : Integrator  InitialCondition=T0_f3
  T_f4 : Integrator  InitialCondition=T0_f4
  T_g1 : Integrator  InitialCondition=T0_g1
  T_g2 : Integrator  InitialCondition=T0_g2
  T_g3 : Integrator  InitialCondition=T0_g3
  To Workspace : ToWorkspace  VariableName=core_ht  SaveFormat=Timeseries  SampleTime=-1
  To Workspace1 : ToWorkspace  VariableName=core_graphite_temp  SaveFormat=Timeseries  SampleTime=-1
  To Workspace2 : ToWorkspace  VariableName=core_fert_temp  SaveFormat=Timeseries  SampleTime=-1
  To Workspace3 : ToWorkspace  VariableName=core_fuel_temp  SaveFormat=Timeseries  SampleTime=-1
  Core Temperatures : Outport  VectorParamsAs1DForOutWhenUnconnected=off
  wires:
  Fuel Heat Transfer Fraction/1 -> [fuel_hA_frac]
  Fuel Flow Fraction/1 -> [fuel_flow_frac]
  Core Power (Frac)/1 -> [Core_Power_frac]
  Fuel Inlet Temperature/1 -> [Tf_in]
  Blanket Inlet Temperature/1 -> [Tb_in]
  Blanket Flow Fraction/1 -> [blank_flow_frac]
  Blanket Heat Transfer Fraction/1 -> [blank_hA_frac]
  T_g1/1 -> Minus/2, Scope/1, [T_g1]
  [Core_Temperatures] -> Core Temperatures/1
  Constant/1 -> [P]
  Constant1/1 -> [hA_fg_up]
  Constant2/1 -> [hA_fg_dn]
  Constant3/1 -> [hA_bg]
  Constant4/1 -> [k_g1]
  Constant5/1 -> [k_g2]
  Constant6/1 -> [mcp_g1]
  Constant7/1 -> [mcp_g2]
  Constant8/1 -> [k_f1]
  Constant9/1 -> [mcp_f1]
  Constant10/1 -> [tau_1]
  Constant11/1 -> [k_1]
  Constant12/1 -> [k_f2]
  Constant13/1 -> [mcp_f2]
  Constant14/1 -> [tau_2]
  Constant15/1 -> [k_2]
  Constant16/1 -> [k_f3]
  Constant17/1 -> [mcp_f3]
  Constant19/1 -> [k_3]
  Constant18/1 -> [tau_3]
  Constant20/1 -> [k_f4]
  Constant21/1 -> [mcp_f4]
  Constant22/1 -> [tau_4]
  Constant23/1 -> [k_4]
  Constant25/1 -> [mcp_g3]
  Constant24/1 -> [k_g3]
  Constant26/1 -> [k_b1]
  Constant27/1 -> [mcp_b1]
  Constant28/1 -> [tau_b1]
  Constant29/1 -> [k_1b]
  Constant30/1 -> [k_b2]
  Constant31/1 -> [mcp_b2]
  Constant32/1 -> [tau_b2]
  Constant33/1 -> [k_2b]
  Mux1/1 -> To Workspace/1
  [Core_Power_frac] -> Mux1/1
  [Tb_in] -> Mux3/1, Fertile Temperature Scope/1, Mux1/3
  [T_g1] -> Mux2/1, Graphite Temperature Scope/1, Mux1/4
  [T_f1] -> Mux1/5, Mux4/2, Fuel Temperature Scope/2
  [T_f2] -> Mux4/3, Fuel Temperature Scope/3, Mux1/6
  [T_g2] -> Mux2/2, Graphite Temperature Scope/2, Mux1/7
  [T_f3] -> Mux4/4, Fuel Temperature Scope/4, Mux1/8
  [T_g3] -> Mux2/3, Graphite Temperature Scope/3, Mux1/10
  [T_b1] -> Mux3/2, Fertile Temperature Scope/2, Mux1/11
  [T_b2] -> Mux3/3, Fertile Temperature Scope/3, Mux1/12
  [fuel_flow_frac] -> Mux1/13
  [fuel_hA_frac] -> Mux1/14
  [blank_flow_frac] -> Mux1/15
  [blank_hA_frac] -> Mux1/16
  [hA_fg_up] -> Divide/1
  [fuel_hA_frac] -> Divide/2
  [mcp_g1] -> Divide/3
  Divide/1 -> Product/1
  Minus/1 -> Product/2
  [T_f1] -> Minus/1
  Product/1 -> Plus/1
  Divide1/1 -> Plus/2
  [Core_Power_frac] -> Divide1/3
  [P] -> Divide1/2
  [k_g1] -> Divide1/1
  [mcp_g1] -> Divide1/4
  Plus/1 -> T_g1/1
  Divide2/1 -> Plus1/1
  Divide3/1 -> Plus1/2
  [Tf_in] -> Plus2/1
  Plus2/1 -> Divide2/1
  [fuel_flow_frac] -> Divide2/2
  [tau_1] -> Divide2/3
  [Core_Power_frac] -> Divide3/3
  [P] -> Divide3/2
  [k_f1] -> Divide3/1
  [mcp_f1] -> Divide3/4
  Divide4/1 -> Plus1/3
  [T_g1] -> Plus3/1
  [mcp_f1] -> Divide4/5
  Plus3/1 -> Divide4/4
  [k_1] -> Divide4/3
  [hA_fg_up] -> Divide4/2
  [fuel_hA_frac] -> Divide4/1
  Plus1/1 -> T_f1/1
  Plus4/1 -> T_f2/1
  [fuel_hA_frac] -> Divide7/1
  [hA_fg_up] -> Divide7/2
  [k_2] -> Divide7/3
  Plus6/1 -> Divide7/4
  [mcp_f2] -> Divide7/5
  [T_g1] -> Plus6/1
  Divide7/1 -> Plus4/3
  [mcp_f2] -> Divide6/4
  [k_f2] -> Divide6/1
  [P] -> Divide6/2
  [Core_Power_frac] -> Divide6/3
  [tau_2] -> Divide5/3
  [fuel_flow_frac] -> Divide5/2
  Plus5/1 -> Divide5/1
  T_f2/1 -> Plus5/2, Scope3/1, [T_f2]
  [T_f1] -> Plus5/1
  Divide6/1 -> Plus4/2
  Divide5/1 -> Plus4/1
  Plus7/1 -> T_g2/1
  [mcp_g2] -> Divide9/4
  [k_g2] -> Divide9/1
  [P] -> Divide9/2
  [Core_Power_frac] -> Divide9/3
  Divide9/1 -> Plus7/2
  Product1/1 -> Plus7/1
  [T_f3] -> Minus1/1
  Minus1/1 -> Product1/2
  Divide8/1 -> Product1/1
  [mcp_g2] -> Divide8/3
  [fuel_hA_frac] -> Divide8/2
  [hA_fg_dn] -> Divide8/1
  T_g2/1 -> Scope1/1, [T_g2], Minus1/2
  Divide13/1 -> Plus11/1
  Divide14/1 -> Plus11/2
  [T_f3] -> Plus12/1
  T_f4/1 -> Scope5/1, [T_f4], Plus12/2
  Plus12/1 -> Divide13/1
  [fuel_flow_frac] -> Divide13/2
  [tau_4] -> Divide13/3
  [Core_Power_frac] -> Divide14/3
  [P] -> Divide14/2
  [k_f4] -> Divide14/1
  [mcp_f4] -> Divide14/4
  Divide15/1 -> Plus11/3
  [T_g2] -> Plus13/1
  [mcp_f4] -> Divide15/5
  Plus13/1 -> Divide15/4
  [k_4] -> Divide15/3
  [hA_fg_dn] -> Divide15/2
  [fuel_hA_frac] -> Divide15/1
  Plus11/1 -> T_f4/1
  Plus8/1 -> T_f3/1
  [fuel_hA_frac] -> Divide12/1
  [hA_fg_dn] -> Divide12/2
  [k_3] -> Divide12/3
  Plus10/1 -> Divide12/4
  [mcp_f3] -> Divide12/5
  [T_g2] -> Plus10/1
  Divide12/1 -> Plus8/3
  [mcp_f3] -> Divide11/4
  [k_f3] -> Divide11/1
  [P] -> Divide11/2
  [Core_Power_frac] -> Divide11/3
  [tau_3] -> Divide10/3
  [fuel_flow_frac] -> Divide10/2
  Plus9/1 -> Divide10/1
  T_f3/1 -> Plus9/2, Plus13/2, Plus10/2, Scope4/1, [T_f3]
  [T_f2] -> Plus9/1
  Divide11/1 -> Plus8/2
  Divide10/1 -> Plus8/1
  Divide16/1 -> Plus19/1
  Divide17/1 -> Plus19/2
  [Tb_in] -> Plus20/1
  T_b1/1 -> Scope6/1, [T_b1], Plus14/2, Plus17/2, Plus20/2
  Plus20/1 -> Divide16/1
  [blank_flow_frac] -> Divide16/2
  [tau_b1] -> Divide16/3
  [Core_Power_frac] -> Divide17/3
  [P] -> Divide17/2
  [k_b1] -> Divide17/1
  [mcp_b1] -> Divide17/4
  Divide18/1 -> Plus19/3
  [T_g3] -> Plus14/1
  [mcp_b1] -> Divide18/5
  Plus14/1 -> Divide18/4
  [k_1b] -> Divide18/3
  [hA_bg] -> Divide18/2
  [blank_hA_frac] -> Divide18/1
  Plus19/1 -> T_b1/1
  Plus15/1 -> T_b2/1
  [blank_hA_frac] -> Divide21/1
  [hA_bg] -> Divide21/2
  [k_2b] -> Divide21/3
  Plus17/1 -> Divide21/4
  [mcp_b2] -> Divide21/5
  [T_g3] -> Plus17/1
  Divide21/1 -> Plus15/3
  [mcp_b2] -> Divide20/4
  [k_b2] -> Divide20/1
  [P] -> Divide20/2
  [Core_Power_frac] -> Divide20/3
  [tau_b2] -> Divide19/3
  [blank_flow_frac] -> Divide19/2
  Plus16/1 -> Divide19/1
  T_b2/1 -> Plus16/2, Scope7/1, [T_b2]
  [T_b1] -> Plus16/1
  Divide20/1 -> Plus15/2
  Divide19/1 -> Plus15/1
  T_g3/1 -> Minus2/2, Scope8/1, [T_g3]
  [hA_bg] -> Divide22/1
  [blank_hA_frac] -> Divide22/2
  [mcp_g3] -> Divide22/3
  Divide22/1 -> Product2/1
  Minus2/1 -> Product2/2
  [T_b1] -> Minus2/1
  Product2/1 -> Plus18/1
  Divide23/1 -> Plus18/2
  [Core_Power_frac] -> Divide23/3
  [P] -> Divide23/2
  [k_g3] -> Divide23/1
  [mcp_g3] -> Divide23/4
  Plus18/1 -> T_g3/1
  [T_b2] -> Mux/9
  [T_b1] -> Mux/8
  [T_g3] -> Mux/7
  [T_f4] -> Mux/6
  [T_f3] -> Mux/5
  [T_g2] -> Mux/4
  [T_f2] -> Mux/3
  [T_f1] -> Mux/2
  [T_g1] -> Mux/1
  Mux/1 -> [Core_Temperatures]
  T_f1/1 -> Scope2/1, [T_f1], Plus3/2, Plus6/2, Plus2/2
  [T_f4] -> Mux1/9, Mux4/5, Fuel Temperature Scope/5
  [Tf_in] -> Fuel Temperature Scope/1, Mux4/1, Mux1/2
  Mux2/1 -> To Workspace1/1
  Mux3/1 -> To Workspace2/1
  Mux4/1 -> To Workspace3/1

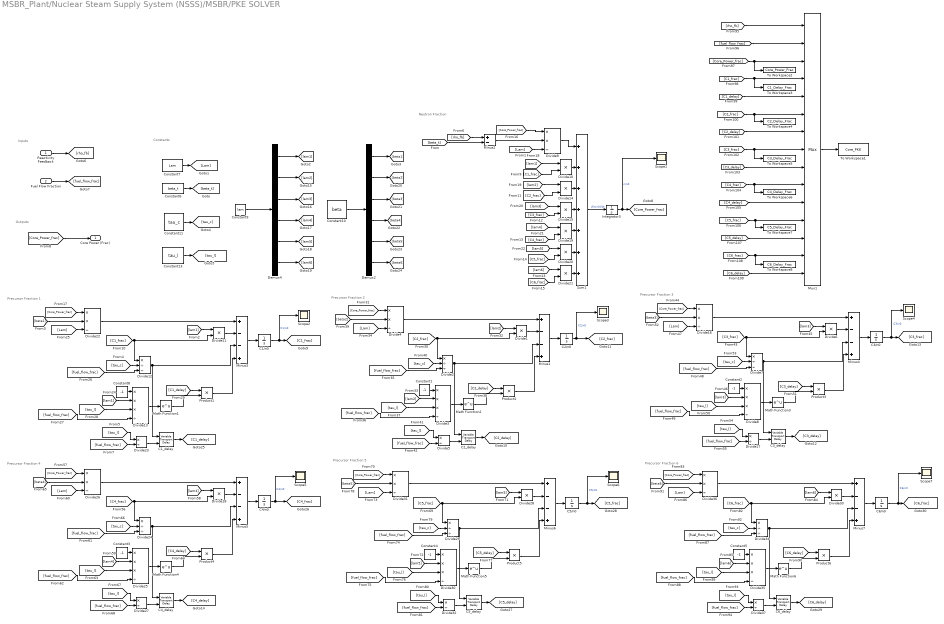
== system MSBR_Plant/Nuclear Steam Supply System (NSSS)/MSBR/PKE SOLVER ==
  note: Precursor Fraction 6
  note: Precursor Fraction 5
  note: Precursor Fraction 4
  note: Precursor Fraction 3
  note: Precursor Fraction 2
  note: Precursor Fraction 1
  note: Neutron Fraction
  note: Constants
  note: Outputs
  note: Inputs
  Reactivity Feedback : Inport
  Fuel Flow Fraction : Inport  Port=2
  C1/n0 : Integrator  InitialCondition=C0(1)
  C1_delay : VariableTransportDelay  MaximumDelay=1000000  InitialOutput=C0(1)/tau_c
  C2/n0 : Integrator  InitialCondition=C0(2)
  C2_delay : VariableTransportDelay  MaximumDelay=1000000  InitialOutput=C0(2)/tau_c
  C3/n0 : Integrator  InitialCondition=C0(3)
  C3_delay : VariableTransportDelay  MaximumDelay=1000000  InitialOutput=C0(3)/tau_c
  C4/n0 : Integrator  InitialCondition=C0(4)
  C4_delay : VariableTransportDelay  MaximumDelay=1000000  InitialOutput=C0(4)/tau_c
  C5/n0 : Integrator  InitialCondition=C0(5)
  C5_delay : VariableTransportDelay  MaximumDelay=1000000  InitialOutput=C0(5)/tau_c
  C6/n0 : Integrator  InitialCondition=C0(6)
  C6_delay : VariableTransportDelay  MaximumDelay=1000000  InitialOutput=C0(6)/tau_c
  Constant{1..5,8} (6 alike) : Constant  Value=-1
  Constant10 : Constant  Value=beta
  Constant11 : Constant  Value=tau_c
  Constant13 : Constant  Value=tau_l
  Constant6 : Constant  Value=beta_t
  Constant7 : Constant  Value=Lam
  Constant9 : Constant  Value=lam
  Demux2 : Demux  Outputs=6
  Demux4 : Demux  Outputs=6
  Divide{1,6,10..11,14..15,18..21,28,33} (12 alike) : Product  Inputs=**
  Divide{2,7,12,24,29,34} (6 alike) : Product  Inputs=*//
  Divide{3,8,13,25,30,35} (6 alike) : Product  Inputs=***/
  Divide{4,9,16,22,26,31,36} (7 alike) : Product  Inputs=**/
  Divide{5,17,23,27,32,37} (6 alike) : Product  Inputs=*/
  Integrator3 : Integrator  InitialCondition=n_frac0
  Math Function{1..6} (6 alike) : Math  SaturateOnIntegerOverflow=on
  Minus{1,3..7} (6 alike) : Sum  Inputs=+--+
  Minus2 : Sum  Inputs=+-
  Mux1 : Mux  Inputs=15
  Product{1..6} (6 alike) : Product
  Scope{1..7} (7 alike) : Scope
  Sum1 : Sum  Inputs=+++++++
  To Workspace1 : ToWorkspace  VariableName=Core_PKE  SaveFormat=Timeseries  SampleTime=-1
  To Workspace2 : ToWorkspace  VariableName=Core_Power_Frac  SaveFormat=Timeseries  SampleTime=-1
  To Workspace3 : ToWorkspace  VariableName=C1_Delay_Frac  SaveFormat=Timeseries  SampleTime=-1
  To Workspace4 : ToWorkspace  VariableName=C2_Delay_Frac  SaveFormat=Timeseries  SampleTime=-1
  To Workspace5 : ToWorkspace  VariableName=C3_Delay_Frac  SaveFormat=Timeseries  SampleTime=-1
  To Workspace6 : ToWorkspace  VariableName=C4_Delay_Frac  SaveFormat=Timeseries  SampleTime=-1
  To Workspace7 : ToWorkspace  VariableName=C5_Delay_Frac  SaveFormat=Timeseries  SampleTime=-1
  To Workspace8 : ToWorkspace  VariableName=C6_Delay_Frac  SaveFormat=Timeseries  SampleTime=-1
  Core Power (Frac) : Outport
  wires:
  Product1/1 -> Minus3/4
  Divide23/1 -> C1_delay/2
  Divide11/1 -> Minus3/2
  Divide12/1 -> Minus3/3, C1_delay/1
  Divide22/1 -> Minus3/1
  Constant11/1 -> [tau_c]
  Divide13/1 -> Math Function1/1
  Divide14/1 -> Sum1/3
  Integrator3/1 -> Scope1/1, [Core_Power_frac]  "n/n0"
  Sum1/1 -> Integrator3/1  "d(n/n0)/dt"
  Minus2/1 -> Divide9/2
  Divide21/1 -> Sum1/7
  Divide20/1 -> Sum1/6
  Minus3/1 -> C1/n0/1
  [beta1] -> Divide22/2
  Divide15/1 -> Sum1/4
  Divide9/1 -> Sum1/1
  Divide10/1 -> Sum1/2
  Math Function1/1 -> Product1/2
  Constant9/1 -> Demux4/1
  Constant10/1 -> Demux2/1
  Divide19/1 -> Sum1/5
  [Lam] -> Divide9/3
  Constant8/1 -> Divide13/1
  Reactivity Feedback/1 -> [rho_fb]
  Constant6/1 -> [beta_t]
  [beta_t] -> Minus2/2
  Constant7/1 -> [Lam]
  [tau_c] -> Divide12/2
  [tau_l] -> Divide23/1
  Constant13/1 -> [tau_l]
  [rho_fb] -> Minus2/1
  [fuel_flow_frac] -> Divide23/2
  Fuel Flow Fraction/1 -> [fuel_flow_frac]
  [Core_Power_frac] -> Core Power (Frac)/1
  [C1_frac] -> Divide10/2
  [C1_frac] -> Divide11/2, Divide12/1
  C1/n0/1 -> Scope2/1, [C1_frac]  "C1/n0"
  [C2_frac] -> Divide14/2
  [C3_frac] -> Divide15/2
  [C4_frac] -> Divide19/2
  [C5_frac] -> Divide20/2
  [C6_frac] -> Divide21/2
  [Core_Power_frac] -> Divide9/1
  [Core_Power_frac] -> Divide22/1
  Demux4/1 -> [lam1]
  Demux4/2 -> [lam2]
  Demux4/3 -> [lam3]
  Demux4/4 -> [lam4]
  Demux4/5 -> [lam5]
  Demux4/6 -> [lam6]
  [lam1] -> Divide10/1
  [lam2] -> Divide14/1
  [lam3] -> Divide15/1
  [lam4] -> Divide19/1
  [lam5] -> Divide20/1
  [lam6] -> Divide21/1
  [lam1] -> Divide11/1
  [lam1] -> Divide13/2
  [Lam] -> Divide22/3
  Demux2/1 -> [beta1]
  Demux2/2 -> [beta2]
  Demux2/3 -> [beta3]
  Demux2/4 -> [beta4]
  Demux2/5 -> [beta5]
  Demux2/6 -> [beta6]
  [fuel_flow_frac] -> Divide12/3
  [fuel_flow_frac] -> Divide13/4
  [tau_l] -> Divide13/3
  C1_delay/1 -> [C1_delay]
  [C1_delay] -> Product1/1
  [C2_delay] -> Product2/1
  C2_delay/1 -> [C2_delay]
  [tau_l] -> Divide3/3
  [fuel_flow_frac] -> Divide3/4
  [fuel_flow_frac] -> Divide2/3
  [Lam] -> Divide4/3
  [lam2] -> Divide3/2
  [lam2] -> Divide1/1
  [Core_Power_frac] -> Divide4/1
  C2/n0/1 -> Scope3/1, [C2_frac]  "C2/n0"
  [C2_frac] -> Divide2/1, Divide1/2
  [fuel_flow_frac] -> Divide5/2
  [tau_l] -> Divide5/1
  [tau_c] -> Divide2/2
  Constant1/1 -> Divide3/1
  Math Function2/1 -> Product2/2
  [beta2] -> Divide4/2
  Minus1/1 -> C2/n0/1
  Divide3/1 -> Math Function2/1
  Divide4/1 -> Minus1/1
  Divide2/1 -> C2_delay/1, Minus1/3
  Divide1/1 -> Minus1/2
  Divide5/1 -> C2_delay/2
  Product2/1 -> Minus1/4
  Product3/1 -> Minus4/4
  Divide17/1 -> C3_delay/2
  Divide6/1 -> Minus4/2
  Divide7/1 -> Minus4/3, C3_delay/1
  Divide16/1 -> Minus4/1
  Divide8/1 -> Math Function3/1
  Minus4/1 -> C3/n0/1
  [beta3] -> Divide16/2
  Math Function3/1 -> Product3/2
  Constant2/1 -> Divide8/1
  [tau_c] -> Divide7/2
  [tau_l] -> Divide17/1
  [fuel_flow_frac] -> Divide17/2
  [C3_frac] -> Divide6/2, Divide7/1
  C3/n0/1 -> Scope4/1, [C3_frac]  "C3/n0"
  [Core_Power_frac] -> Divide16/1
  [lam3] -> Divide6/1
  [lam3] -> Divide8/2
  [Lam] -> Divide16/3
  [fuel_flow_frac] -> Divide7/3
  [fuel_flow_frac] -> Divide8/4
  [tau_l] -> Divide8/3
  C3_delay/1 -> [C3_delay]
  [C3_delay] -> Product3/1
  [C4_delay] -> Product4/1
  C4_delay/1 -> [C4_delay]
  [tau_l] -> Divide25/3
  [fuel_flow_frac] -> Divide25/4
  [fuel_flow_frac] -> Divide24/3
  [Lam] -> Divide26/3
  [lam4] -> Divide25/2
  [lam4] -> Divide18/1
  [Core_Power_frac] -> Divide26/1
  C4/n0/1 -> Scope5/1, [C4_frac]  "C4/n0"
  [C4_frac] -> Divide24/1, Divide18/2
  [fuel_flow_frac] -> Divide27/2
  [tau_l] -> Divide27/1
  [tau_c] -> Divide24/2
  Constant3/1 -> Divide25/1
  Math Function4/1 -> Product4/2
  [beta4] -> Divide26/2
  Minus5/1 -> C4/n0/1
  Divide25/1 -> Math Function4/1
  Divide26/1 -> Minus5/1
  Divide24/1 -> C4_delay/1, Minus5/3
  Divide18/1 -> Minus5/2
  Divide27/1 -> C4_delay/2
  Product4/1 -> Minus5/4
  Product5/1 -> Minus6/4
  Divide32/1 -> C5_delay/2
  Divide28/1 -> Minus6/2
  Divide29/1 -> Minus6/3, C5_delay/1
  Divide31/1 -> Minus6/1
  Divide30/1 -> Math Function5/1
  Minus6/1 -> C5/n0/1
  [beta5] -> Divide31/2
  Math Function5/1 -> Product5/2
  Constant4/1 -> Divide30/1
  [tau_c] -> Divide29/2
  [tau_l] -> Divide32/1
  [fuel_flow_frac] -> Divide32/2
  [C5_frac] -> Divide28/2, Divide29/1
  C5/n0/1 -> Scope6/1, [C5_frac]  "C5/n0"
  [Core_Power_frac] -> Divide31/1
  [lam5] -> Divide28/1
  [lam5] -> Divide30/2
  [Lam] -> Divide31/3
  [fuel_flow_frac] -> Divide29/3
  [fuel_flow_frac] -> Divide30/4
  [tau_l] -> Divide30/3
  C5_delay/1 -> [C5_delay]
  [C5_delay] -> Product5/1
  [C6_delay] -> Product6/1
  C6_delay/1 -> [C6_delay]
  [tau_l] -> Divide35/3
  [fuel_flow_frac] -> Divide35/4
  [fuel_flow_frac] -> Divide34/3
  [Lam] -> Divide36/3
  [lam6] -> Divide35/2
  [lam6] -> Divide33/1
  [Core_Power_frac] -> Divide36/1
  C6/n0/1 -> Scope7/1, [C6_frac]  "C6/n0"
  [C6_frac] -> Divide34/1, Divide33/2
  [fuel_flow_frac] -> Divide37/2
  [tau_l] -> Divide37/1
  [tau_c] -> Divide34/2
  Constant5/1 -> Divide35/1
  Math Function6/1 -> Product6/2
  [beta6] -> Divide36/2
  Minus7/1 -> C6/n0/1
  Divide35/1 -> Math Function6/1
  Divide36/1 -> Minus7/1
  Divide34/1 -> C6_delay/1, Minus7/3
  Divide33/1 -> Minus7/2
  Divide37/1 -> C6_delay/2
  Product6/1 -> Minus7/4
  [rho_fb] -> Mux1/1
  [fuel_flow_frac] -> Mux1/2
  [Core_Power_frac] -> To Workspace2/1, Mux1/3
  [C1_frac] -> To Workspace3/1, Mux1/4
  [C1_delay] -> Mux1/5
  [C2_frac] -> To Workspace4/1, Mux1/6
  [C2_delay] -> Mux1/7
  [C3_frac] -> To Workspace5/1, Mux1/8
  [C3_delay] -> Mux1/9
  [C4_frac] -> To Workspace6/1, Mux1/10
  [C4_delay] -> Mux1/11
  [C5_frac] -> To Workspace7/1, Mux1/12
  [C5_delay] -> Mux1/13
  [C6_frac] -> To Workspace8/1, Mux1/14
  [C6_delay] -> Mux1/15
  Mux1/1 -> To Workspace1/1
